simulink model "sistemaLazoAbiertoNoLineal"  (R2012b)
settings: Solver=ode45  StartTime=0.0  StopTime=8  RelTol=1e-3
values from neighbouring files (symbols this model uses):
  b_m = bm+(bl/r^2)    (= 1.5e-05)    [InicializaYconstantes.m]
  J_m = Jm+(Jl/r^2)    (= 5.65099476805e-06)    [InicializaYconstantes.m]
  lambda = 0.01546    [InicializaYconstantes.m]
  Ld = 6.6*10^-3    (= 0.0066)    [InicializaYconstantes.m]
  Lq = 5.8*10^-3    (= 0.0058)    [InicializaYconstantes.m]
  Pp = 3    [InicializaYconstantes.m]
  Rs = 1.02    [InicializaYconstantes.m]
  T_l = Tl/r    (= 0.00499521477515)    [InicializaYconstantes.m]
settings Model: Creator=usuario  LastModifiedBy=usuario

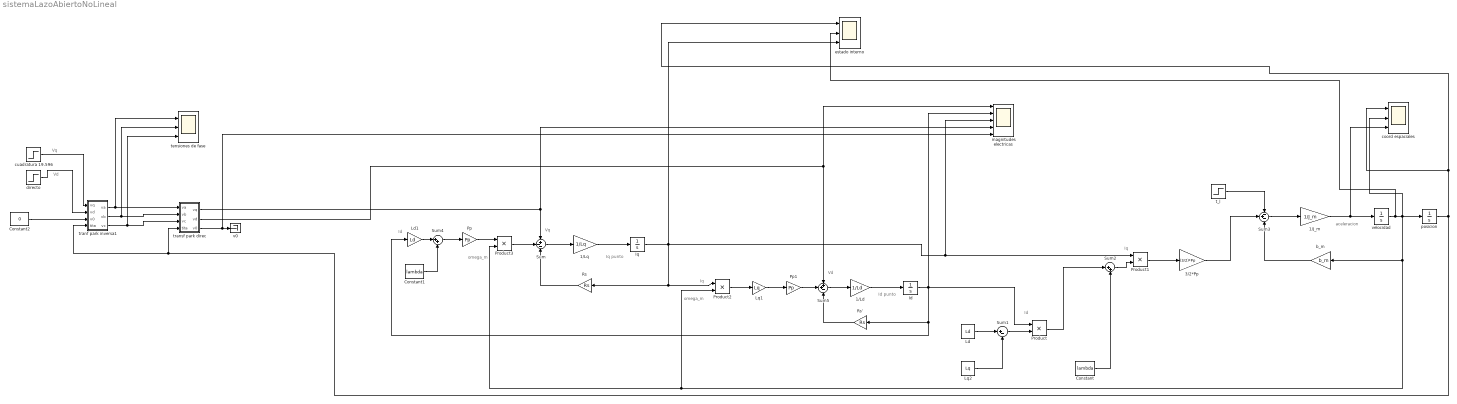
== system sistemaLazoAbiertoNoLineal ==
  note: Vd
  note: Vq
  note: Vd
  note: omega_m
  note: Iq
  note: Id punto
  note: Vq
  note: Id
  note: Iq punto
  note: Iq
  note: aceleracion
  note: Id
  note: omega_m
  1/J_m : Gain  Gain=1/J_m
  1/Ld : Gain  Gain=1/Ld
  1/Lq : Gain  Gain=1/Lq
  3/2*Pp : Gain  Gain=(3/2)*Pp
  Constant : Constant  Value=lambda
  Constant1 : Constant  Value=lambda
  Constant2 : Constant  Value=0
  Id : Integrator
  Iq : Integrator
  Ld : Constant  Value=Ld
  Ld1 : Gain  Gain=Ld
  Lq1 : Gain  Gain=Lq
  Lq2 : Constant  Value=Lq
  Pp : Gain  Gain=Pp
  Pp1 : Gain  Gain=Pp
  Product{,1..3} (4 alike) : Product  RndMeth=Zero
  Rs : Gain  Gain=Rs
  Rs' : Gain  Gain=Rs
  Sum : Sum  Inputs=+--
  Sum1 : Sum  Inputs=|+-
  Sum2 : Sum  Inputs=|++
  Sum3 : Sum  Inputs=-+-
  Sum4 : Sum  Inputs=|++
  Sum5 : Sum  Inputs=++-
  b_m : Gain  Gain=b_m
  coord espaciales : Scope  NumInputPorts=3
      settings: TimeRange=12  YMin=-1000~0~-50000  YMax=3000~300~100000  MaxDataPoints=8000
  cuadratura 19.596 : Step  Time=0.1  After=19.596  SampleTime=0
  directo : Step  After=0  SampleTime=0
  estado interno : Scope  NumInputPorts=3
      settings: TimeRange=8  YMin=-1000~0~-5  YMax=3000~400~10  MaxDataPoints=8000
  magnitudes electricas : Scope  NumInputPorts=5
      settings: TimeRange=8  YMin=-1~-3.567183402155509e-28~-10~0~-1  YMax=1~10~10~20~1  SaveName=ScopeData2  MaxDataPoints=8000
  posicion : Integrator
  t_l : Step  Time=0.3  After=T_l  SampleTime=0
  tensiones de fase : Scope  NumInputPorts=3
      settings: TimeRange=8  YMin=-1000~0~-5  YMax=3000~400~10  SaveName=ScopeData3  MaxDataPoints=8000
  tranf park inversa1 : Subsystem
  transf park direc : Subsystem
  v0 : Terminator
  velocidad : Integrator  ContinuousStateAttributes='velocidad'
  wires:
  Ld/1 -> Sum1/1
  Lq2/1 -> Sum1/2
  Sum1/1 -> Product/2
  Product/1 -> Sum2/1
  Constant/1 -> Sum2/2
  Sum2/1 -> Product1/2
  t_l/1 -> Sum3/1
  Product1/1 -> 3/2*Pp/1
  b_m/1 -> Sum3/3
  Sum3/1 -> 1/J_m/1
  1/Lq/1 -> Iq/1
  1/Ld/1 -> Id/1
  Ld1/1 -> Sum4/1
  Constant1/1 -> Sum4/2
  Sum4/1 -> Pp/1
  Sum/1 -> 1/Lq/1
  Rs/1 -> Sum/3
  cuadratura 19.596/1 -> tranf park inversa1/1(vq)
  Rs'/1 -> Sum5/3
  Lq1/1 -> Pp1/1
  Product2/1 -> Lq1/1
  Iq/1 -> estado interno/3, magnitudes electricas/3, Product1/1, Rs/1, Product2/1
  Sum5/1 -> 1/Ld/1
  Pp1/1 -> Sum5/2
  directo/1 -> tranf park inversa1/2(vd)
  Id/1 -> Rs'/1, Ld1/1, Product/1, magnitudes electricas/2
  3/2*Pp/1 -> Sum3/2
  1/J_m/1 -> coord espaciales/3, velocidad/1
  Pp/1 -> Product3/1
  Product3/1 -> Sum/2
  velocidad/1 -> coord espaciales/2, Product2/2, Product3/2, b_m/1, posicion/1, estado interno/2
  posicion/1 -> tranf park inversa1/4(tita), transf park direc/4(tita), estado interno/1, coord espaciales/1
  tranf park inversa1/1(va) -> tensiones de fase/1, transf park direc/1(va)
  tranf park inversa1/2(vb) -> tensiones de fase/2, transf park direc/2(vb)
  tranf park inversa1/3(vc) -> tensiones de fase/3, transf park direc/3(vc)
  Constant2/1 -> tranf park inversa1/3(v0)
  transf park direc/1(vq) -> Sum/1, magnitudes electricas/4
  transf park direc/2(vd) -> magnitudes electricas/1, Sum5/1
  transf park direc/3(v0) -> magnitudes electricas/5, v0/1

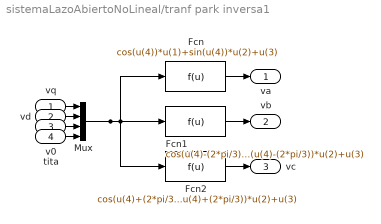
== system sistemaLazoAbiertoNoLineal/tranf park inversa1 ==
  vq : Inport
  vd : Inport  Port=2
  v0 : Inport  Port=3
  tita : Inport  Port=4
  Fcn : Fcn  Expr=cos(u(4))*u(1)+sin(u(4))*u(2)+u(3)
  Fcn1 : Fcn  Expr=cos(u(4)-(2*pi/3))*u(1)+sin(u(4)-(2*pi/3))*u(2)+u(3)
  Fcn2 : Fcn  Expr=cos(u(4)+(2*pi/3))*u(1)+sin(u(4)+(2*pi/3))*u(2)+u(3)
  Mux : Mux
  va : Outport
  vb : Outport  Port=2
  vc : Outport  Port=3
  wires:
  Mux/1 -> Fcn1/1, Fcn/1, Fcn2/1
  Fcn/1 -> va/1
  vq/1 -> Mux/1
  vd/1 -> Mux/2
  Fcn1/1 -> vb/1
  v0/1 -> Mux/3
  tita/1 -> Mux/4
  Fcn2/1 -> vc/1

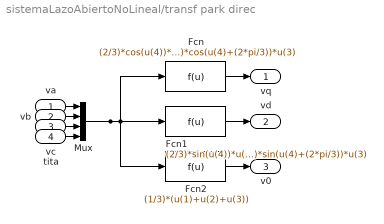
== system sistemaLazoAbiertoNoLineal/transf park direc ==
  va : Inport
  vb : Inport  Port=2
  vc : Inport  Port=3
  tita : Inport  Port=4
  Fcn : Fcn  Expr=(2/3)*cos(u(4))*u(1)+(2/3)*cos(u(4)-(2*pi/3))*u(2)+(2/3)*cos(u(4)+(2*pi/3))*u(3)
  Fcn1 : Fcn  Expr=(2/3)*sin(u(4))*u(1)+(2/3)*sin(u(4)-(2*pi/3))*u(2)+(2/3)*sin(u(4)+(2*pi/3))*u(3)
  Fcn2 : Fcn  Expr=(1/3)*(u(1)+u(2)+u(3))
  Mux : Mux
  vq : Outport
  vd : Outport  Port=2
  v0 : Outport  Port=3
  wires:
  Mux/1 -> Fcn1/1, Fcn/1, Fcn2/1
  Fcn/1 -> vq/1
  va/1 -> Mux/1
  vb/1 -> Mux/2
  Fcn1/1 -> vd/1
  vc/1 -> Mux/3
  tita/1 -> Mux/4
  Fcn2/1 -> v0/1
